simulink model "First_order_system_CS"  (R2023b)
settings: Solver=VariableStepAuto  StartTime=0.0  StopTime=100  RelTol=1e-3
settings Model: Creator=devan  LastModifiedBy=devan

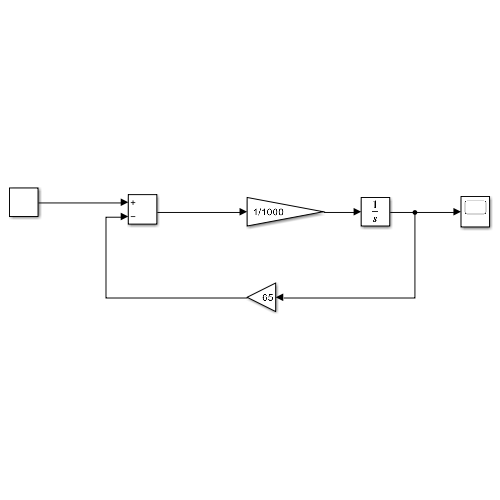
[thumbnail: Simulink's stored preview of the top-level diagram]
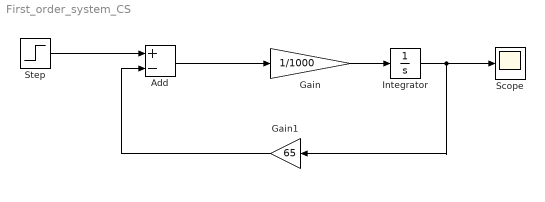
== system First_order_system_CS ==
  Add : Sum  Inputs=+-
  Gain : Gain  Gain=1/1000
  Gain1 : Gain  Gain=65
  Integrator : Integrator
  Scope : Scope
  Step : Step  Time=3  SampleTime=0
  wires:
  Add/1 -> Gain/1
  Gain/1 -> Integrator/1
  Integrator/1 -> Gain1/1, Scope/1
  Step/1 -> Add/1
  Gain1/1 -> Add/2
